simulink model "verify_Heat_Capacity2_mdl"  (R2013b)
settings: Solver=ode45  StartTime=0.0  StopTime=5  RelTol=1e-3
libraries: carnot x2, simulink x1
settings Model: Creator=darl  LastModifiedBy=drhf
settings DataIOCC: LimitDataPoints=off
settings DebuggingCC: UnderspecifiedInitializationDetection=Simplified  MergeDetectMultiDrivingBlocksExec=error  SolverPrmCheckMsg=none  FrameProcessingCompatibilityMsg=error
settings HardwareCC: ProdBitPerPointer=64  ProdLargestAtomicFloat=Float  ProdIntDivRoundTo=Zero  ProdEndianess=LittleEndian  ProdHWDeviceType=Specified
settings ModelReferenceCC: PropagateSignalLabelsOutOfModel=on
settings GRTTargetCC: CodeReplacementLibrary=C89/C90 (ANSI)  GeneratePreprocessorConditionals=Use local settings

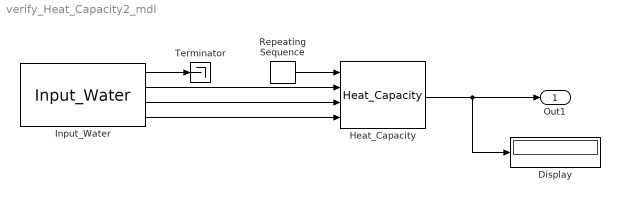
== system verify_Heat_Capacity2_mdl ==
  Display : Display
  Heat_Capacity : carnot/Basic/Material_Properties/Heat_Capacity  VariantControl=CarlibClassic  INPUTARGUMENTS=state variables (classic)  DEBUGLEVEL=DEBUGLEVEL  MAXTOTALWARNINGS=inf  MAXCONSECUTIVEWARNINGS=inf  WRITETOFILE=0  FILENAME='errors.txt'
  Input_Water : carnot/Basic/Material_Properties/Input_Water  T=20  p=2e6  xd=0
  Repeating Sequence : simulink/Sources/Repeating Sequence  rep_seq_t=0:6  rep_seq_y=[0.01 4.44 10 15.6 21.1 26.7 32.2]
  Terminator : Terminator
  Out1 : Outport
  wires:
  Input_Water/4 -> Heat_Capacity/4
  Input_Water/3 -> Heat_Capacity/3
  Input_Water/2 -> Heat_Capacity/2
  Input_Water/1 -> Terminator/1
  Repeating Sequence/1 -> Heat_Capacity/1
  Heat_Capacity/1 -> Display/1, Out1/1
